simulink model "Lidar"  (R2022b)
settings: Solver=FixedStepAuto  StartTime=0.0  StopTime=inf  FixedStep=Ts  RelTol=1e-3
InitFcn:
  | Ts=0.01;
undefined symbols (not defined in the file or in its folder): angle_increment, angle_max, angle_min, data, ranges
libraries: ros2lib x2, instrumentseriallib x2, simulink x1
settings Model: Creator=System-10  LastModifiedBy=System-10

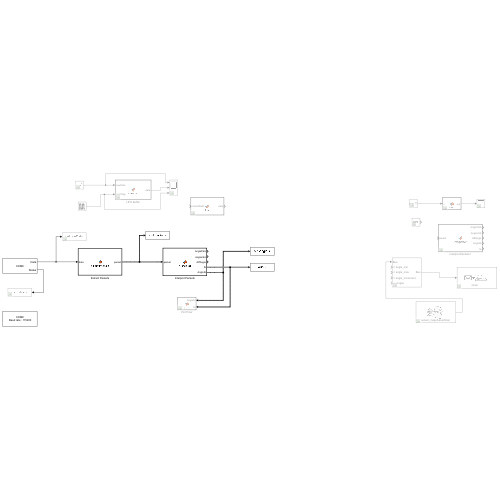
[thumbnail: Simulink's stored preview of the top-level diagram]
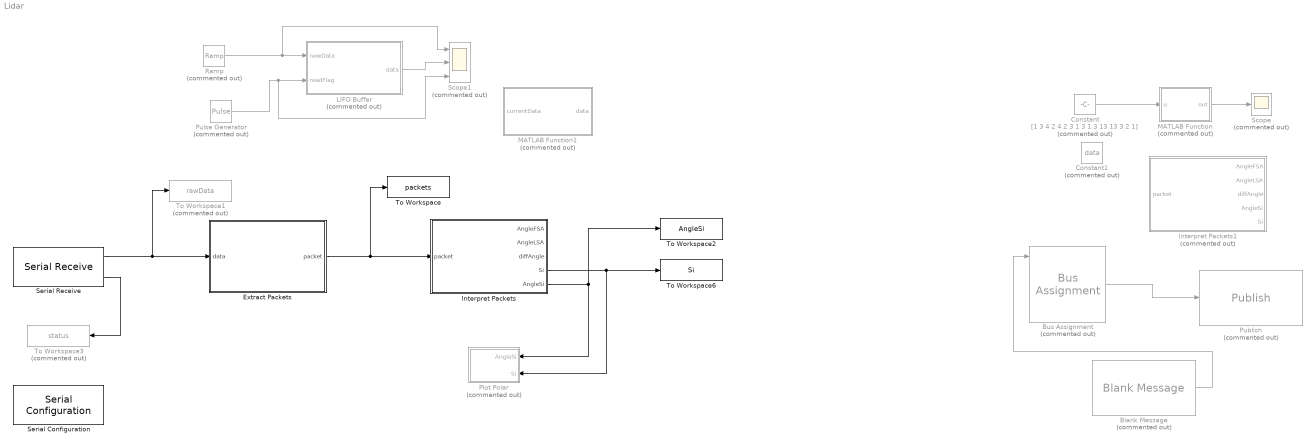
== system Lidar ==
  Blank Message : ros2lib/Blank Message  Commented=on  messageClass=Message  entityType=sensor_msgs/LaserScan  messageType=sensor_msgs/LaserScan  SampleTime=0.1
      settings: LibrarySourceBlock=roslib/ROS 2/Blank Message
  Bus Assignment : BusAssignment  Commented=on  AssignedSignals=angle_min,angle_max,angle_increment,ranges
  Constant : Constant  Commented=on  Value=[1 3 4 2 4 2 3 1 3 1 3 13 13 3 2 1]
  Constant1 : Constant  Commented=on  Value=data  VectorParams1D=off
  Extract Packets : MATLAB Function  TreatAsAtomicUnit=on
  Interpret Packets : MATLAB Function  TreatAsAtomicUnit=on
  Interpret Packets1 : MATLAB Function  Commented=on  TreatAsAtomicUnit=on
  LIFO Buffer : MATLAB Function  Commented=on  TreatAsAtomicUnit=on
  MATLAB Function : MATLAB Function  Commented=on  TreatAsAtomicUnit=on
  MATLAB Function1 : MATLAB Function  Commented=on  TreatAsAtomicUnit=on
  Plot Polar : MATLAB Function  Commented=on  TreatAsAtomicUnit=on
  Publish : ros2lib/Publish  Commented=on  topicSource=Specify your own  topic=/scan  messageType=sensor_msgs/LaserScan  QOSHistory=Keep last  QOSDepth=1  QOSReliability=Reliable  QOSDurability=Volatile
      settings: LibrarySourceBlock=roslib/ROS 2/Publish
  Pulse Generator : DiscretePulseGenerator  Commented=on  PulseType=Time based  PulseWidth=5  PhaseDelay=2
  Ramp : simulink/Sources/Ramp  Commented=on  slope=1  start=0  InitialOutput=0
  Scope : Scope  Commented=on
  Scope1 : Scope  Commented=on  NumInputPorts=3
  Serial Configuration : instrumentseriallib/Serial Configuration  Priority=-200000  PortSel=COM9  Port=COM9  ComPort=COM9  BaudRate=115200  DataBits=8  Parity=none  StopBits=1  ByteOrder=little-endian  FlowControl=none  Timeout=10  SimulateUsing=Interpreted execution  BlockInModel=on  aMode=1
  Serial Receive : instrumentseriallib/Serial Receive  Priority=1  PortSel=COM9  Port=COM9  ComPort=COM9  DataType=uint8  SaveDataType=uint8  ToggleHeader=off  Header=[170 85]  ToggleTerminator=off  Terminator=<none>  CustomTerminator=[]  InputFormat=Column major  ToggleDataSize=on  DataSize=[1 2000]  EnableBlockingMode=off  ActionDataUnavailable=Output last received value  ActionWhenDataUnavailable=Output last received value  CustomValue=111  SampleTime=Ts  SimulateUsing=Interpreted execution  BlockInModel=on  aMode=1
  To Workspace : ToWorkspace  VariableName=packets  SaveFormat=Timeseries  SampleTime=-1
  To Workspace1 : ToWorkspace  Commented=on  VariableName=rawData  SaveFormat=Structure  SampleTime=-1
      settings: Save2DSignal=2-D array (concatenate along first dimension)
  To Workspace2 : ToWorkspace  VariableName=AngleSi  SaveFormat=Timeseries  SampleTime=-1
  To Workspace3 : ToWorkspace  Commented=on  VariableName=status  SaveFormat=Structure  SampleTime=-1
      settings: Save2DSignal=2-D array (concatenate along first dimension)
  To Workspace6 : ToWorkspace  VariableName=Si  SaveFormat=Timeseries  SampleTime=-1
  wires:
  MATLAB Function/1(out) -> Scope/1
  Constant/1 -> MATLAB Function/1(u)
  Blank Message/1 -> Bus Assignment/1
  Bus Assignment/1 -> Publish/1
  LIFO Buffer/1(data) -> Scope1/2
  Ramp/1 -> LIFO Buffer/1(newData), Scope1/1
  Pulse Generator/1 -> LIFO Buffer/2(readFlag), Scope1/3
  Serial Receive/1 -> Extract Packets/1(data), To Workspace1/1
  Serial Receive/2 -> To Workspace3/1
  Extract Packets/1(packet) -> Interpret Packets/1(packet), To Workspace/1
  Interpret Packets/4(Si) -> To Workspace6/1, Plot Polar/2(Si)
  Interpret Packets/5(AngleSi) -> Plot Polar/1(AngleSi), To Workspace2/1

== matlab function Lidar/Extract Packets ==
  data: data input; packet output double size=[100 100]
function packet = extractPackets(data)
    persistent indicesOfHeaders;
    persistent packets;
    persistent idx;
    persistent lastData;

    if isempty(lastData)
        lastData = uint8(zeros(1,size(data,2)));
    end

    if isempty(indicesOfHeaders) || ~isequal(data, lastData)
        
        
        indicesOfAA = find(data == 170);
        indicesOfHeaders = zeros(1, length(indicesOfAA)); 
        count = 0;

        for i = 1:length(indicesOfAA)
            if indicesOfAA(i) < length(data) && data(indicesOfAA(i) + 1) == 85
                count = count + 1;
                indicesOfHeaders(count) = indicesOfAA(i);
            end
        end

        indicesOfHeaders = indicesOfHeaders(1:count);

        packets = {};
        idx = 1;
        lastData = data;
        
        for i = 1:length(indicesOfHeaders)-1
            startIdx = indicesOfHeaders(i);
            endIdx = indicesOfHeaders(i+1);
            packets{end+1} = data(startIdx:endIdx-1);
        end
    end
    
    if idx <= length(packets)
        packet = double(packets{idx});
        idx = idx + 1;
    else
        packet = [];
        packets = {};
    end
end

== matlab function Lidar/Interpret Packets ==
  settings: sampleTime=0.01
  data: packet input; AngleFSA output size=[1 100]; AngleLSA output size=[1 100]; diffAngle output size=[1 100]; Si output size=[1 1000]; AngleSi output size=[1 1000]
function [AngleFSA, AngleLSA, diffAngle, Si, AngleSi] = interpreter(packet)
    persistent packets;
    persistent idx;
    
    if isempty(packets)
        packets = {packet};
        idx = 1;
    else
        packets{end+1} = packet;
    end
    
    if idx <= length(packets)
        currentPacket = packets{idx};
        idx = idx + 1;
    else
        AngleFSA = [];
        AngleLSA = [];
        diffAngle = [];
        AngleSi = [];
        Si = [];
        return;
    end
    
    AngleFSA = [];
    AngleLSA = [];
    diffAngle = [];
    AngleSi = [];
    Si = [];

    if size(currentPacket, 2) < 12
        return;
    end

    LSN = currentPacket(1, 4);
    if LSN <= 0
        return;
    end
    
    FSA = bitor(bitshift(uint16(currentPacket(1, 6)), 8), uint16(currentPacket(1, 5)), 'uint16');
    LSA = bitor(bitshift(uint16(currentPacket(1, 8)), 8), uint16(currentPacket(1, 7)), 'uint16');
   
    AngleFSA = double(bitshift(FSA, -1) / 64);
    AngleLSA = double(bitshift(LSA, -1) / 64);
    diffAngle = AngleLSA - AngleFSA;
    
    rawSi = uint8(currentPacket(:, 11:end));
    if mod(size(rawSi, 2), 2)
        return;
    end

    Si = zeros(1, size(rawSi, 2) / 2);
    for i = 1:2:length(rawSi)
        Si((i + 1) / 2) = double(bitor(bitshift(uint16(currentPacket(1, i + 1)), 8), uint16(currentPacket(1, i)), 'uint16'));
    end
    
    AngleSi = zeros(1, LSN);
    AngleSi(1) = AngleFSA;
    for i = 2:LSN - 1
        AngleSi(i) = (diffAngle / (LSN - 1)) * (i - 1) + AngleFSA;
    end
    AngleSi(LSN) = AngleLSA;
    
    % The unit is meter
    Si = Si / 4000; 
    hold on;
end

== matlab function Lidar/Plot Polar ==
  settings: sampleTime=0.01
  data: AngleSi input; Si input
function plot(AngleSi, Si)
    persistent AngleSiHistory SiHistory;
    
    if isempty(AngleSiHistory)
        AngleSiHistory = [];
        SiHistory = [];
    end
    
    if (size(AngleSi) == size(Si))
        AngleSiHistory = [AngleSiHistory, AngleSi];
        SiHistory = [SiHistory, Si];
        
        if size(AngleSiHistory, 2) > 150
            AngleSiHistory = AngleSiHistory(:,end-149:end);
            SiHistory = SiHistory(:,end-149:end);
        end
        
        AngleSiFlat = AngleSiHistory(:);
        SiFlat = SiHistory(:);
        
        polarplot(deg2rad(AngleSiFlat), SiFlat, 'r.', 'MarkerSize', 1);
    else
        return;
    end
end

== matlab function Lidar/MATLAB Function ==
  settings: updateMethod=DISCRETE  sampleTime=1
  data: u input; out output size=[1 20]
function out = func(u)
    persistent indices;
    persistent idx;
    
    if isempty(indices)
        indices = find(u == 1);
        idx = 1;
    end
    
    if idx <= length(indices)
        out = indices(idx);
        idx = idx + 1;
    else
        out = []; % No more indices to output
    end
end

== matlab function Lidar/Interpret Packets1 ==
  settings: updateMethod=DISCRETE  sampleTime=Ts
  data: packet input; AngleFSA output size=[1 100]; AngleLSA output size=[1 100]; diffAngle output size=[1 100]; AngleSi output size=[1 1000]; Si output size=[1 1000]
function [AngleFSA,AngleLSA,diffAngle,AngleSi,Si] = interpreter(packet)

    AngleFSA = [];
    AngleLSA = [];
    diffAngle = [];
    AngleSi = [];
    Si = [];

    if size(packet,2) < 20
        return;
    end

    LSN = packet(1,4);
    if LSN <= 0
        return;
    end
    
    FSA = bitor(bitshift(uint16(packet(1,6)), 8), uint16(packet(1,5)),'uint16');
    
    LSA = bitor(bitshift(uint16(packet(1,8)), 8), uint16(packet(1,7)),'uint16');
    
    %Calculate the Angles
    AngleFSA = double(bitshift(FSA,-1)/64);
    AngleLSA = double(bitshift(LSA,-1)/64);
    diffAngle = AngleLSA - AngleFSA;
    
    rawSi = uint8(packet(:,11:end));
    if mod(size(rawSi,2),2)
        return;
    end

    Si = zeros(1, size(rawSi, 2) / 2);
    for i = 1:2:length(rawSi)
        Si((i+1)/2) = double(bitor(bitshift(uint16(packet(1,i+1)), 8), uint16(packet(1,i)),'uint16'));
    end
    
    AngleSi = zeros(1,LSN);
    AngleSi(1) = AngleFSA;
    for i = 2:LSN-1
        AngleSi(i) = (diffAngle/(LSN-1))*(i - 1)+AngleFSA;
    end
    AngleSi(LSN) = AngleLSA;
    
    %The unit is meter
    Si = Si/4000; 

end

== matlab function Lidar/LIFO Buffer ==
  data: newData input; data output; readFlag input
function data = lifoBuffer(newData, readFlag)
    persistent stack;
    
    if isempty(stack)
        stack = zeros(1,size(newData,2));
    end
    
    if readFlag
        if ~isempty(stack)
            data = stack{end};
            stack(end) = [];
        else
            data = NaN; % or some default value indicating no data
        end
    else
        stack{end+1} = newData;
        data = [];
    end
end

== matlab function Lidar/MATLAB Function1 ==
  data: currentData input; data output size=[1 1000]
function data = fcn(currentData)
    persistent lastData

    if isempty(lastData)
        lastData = uint8(zeros(1,size(currentData,2)));
    end

    if ~(currentData == lastData) 
        lastData = currentData;
        data = double(currentData);
    else
        data = NaN;
    end
end
